simulink model "prob_15b"  (R2015a)
settings: Solver=ode45  StartTime=0.0  StopTime=24  RelTol=1e-3
settings Model: Creator=Anu  LastModifiedBy=Anu

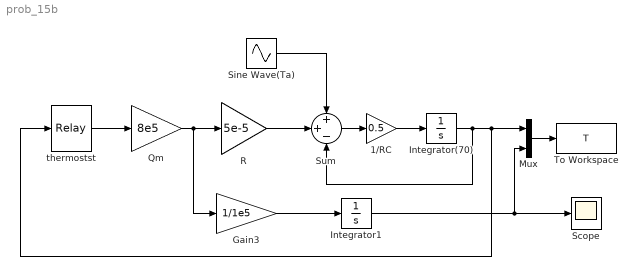
== system prob_15b ==
  1/RC : Gain  Gain=0.5
  Gain3 : Gain  Gain=1/1e5
  Integrator(70) : Integrator  InitialCondition=70
  Integrator1 : Integrator
  Mux : Mux  Inputs=2
  "Qm " : Gain  Gain=8e5
  R : Gain  Gain=5e-5
  Scope : Scope
  Sine Wave(Ta) : Sin  Amplitude=10  Bias=50  Frequency=pi/12  SampleTime=0
  Sum : Sum  Inputs=++-
  To Workspace : ToWorkspace  VariableName=T  SaveFormat=Timeseries  SampleTime=-1
  "thermostst " : Relay  OnSwitchValue=71  OffSwitchValue=69  OnOutputValue=0  OffOutputValue=1
  wires:
  "thermostst "/1 -> "Qm "/1
  Sum/1 -> 1/RC/1
  1/RC/1 -> Integrator(70)/1
  Integrator(70)/1 -> Sum/3, Mux/1, "thermostst "/1
  Sine Wave(Ta)/1 -> Sum/1
  "Qm "/1 -> R/1, Gain3/1
  R/1 -> Sum/2
  Gain3/1 -> Integrator1/1
  Integrator1/1 -> Mux/2, Scope/1
  Mux/1 -> To Workspace/1
